simulink model "RL_TTS1_Controller_6E8X0_Ez_Test(9)"  (R2019b)
settings: Solver=VariableStepAuto  StartTime=0.0  StopTime=100  RelTol=1e-3
PostLoadFcn:
  | if any(exist('dsrtsu_mdlpostloadfcn', 'file') ~= 0), dsrtsu_mdlpostloadfcn('Execute', bdroot); end
undefined symbols (not defined in the file or in its folder): valve_position
libraries: simulink x5
settings Model: DSRTSU_INTERNAL_RTI_VER=550  DSRTSU_INTERNAL_RTI_TYPE=rti1104  RTICANMMDATA=struct('GeneralSetupData',struct('modelroot',['G:\RemoteLabs\RL git repos\Three Tank System set-up\dynamics-and-process-control-6e8x0\Teacher_files'],'generalsettings',struct('filesettings',struct('destfolder',struct('Name','RTICANMM_FILES','Check',1),'buildfolder',struct('Name','.','Check',1),'AbsDestfolder',struct('Name',['G:\RemoteLabs\RL git repos\Three Tank System set-up\dynamics-and-process-control-6e8x0\Teacher_files\RTICANMM_FILES']),'AbsBuildfolder',struct('Name',['G:\RemoteLabs\RL git repos\Three Tank System set-up\dynamics-and-process-control-6e8x0\Teacher_files']))),'options',struct('addpaths',1,'rmpaths',1,'addtrcexclusion',true,'cannavigator',struct('checkmonitoring',0),'show_usrtrc',0,'use_usrtrc',0),'advanced',struct('options',ones(1,100)),'MPSetup',{{}},'RTI',struct('Type','GRT','Ver','','Date',''),'modelname','RL_TTS1_Controller','block','RL_TTS1_Controller'))  DSRTSU_INTERNAL_RTIFPGA=150  Creator=whendrix  LastModifiedBy=20191255
settings SFSimCC: CustomCodeUndefinedFunction=UseInterfaceOnly

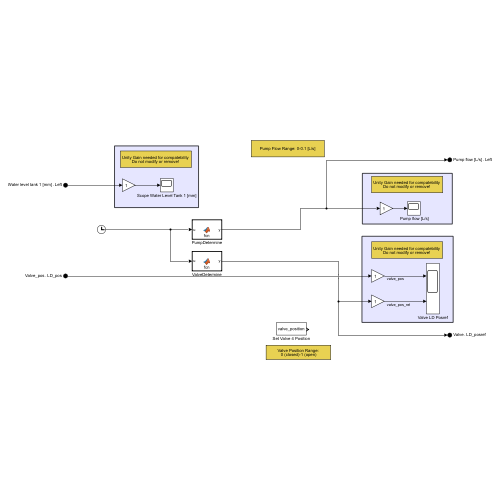
[thumbnail: Simulink's stored preview of the top-level diagram]
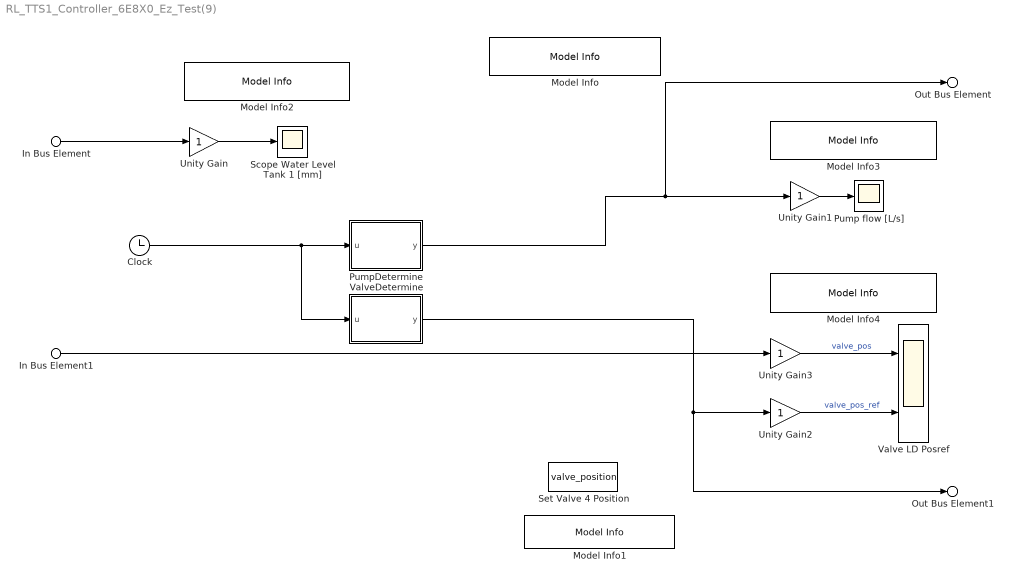
== system RL_TTS1_Controller_6E8X0_Ez_Test(9) ==
  In Bus Element : Inport  PortName=Water level tank 1 [mm]  Element=Left
  In Bus Element1 : Inport  Port=2  PortName=Valve_pos  Element=LD_pos
  " Pump flow [L/s]" : Scope
  Clock : Clock
  Model Info : simulink/Model-Wide Utilities/Model Info  Frame=on  DisplayStringWithTags=Pump Flow Range: 0-0.1 [L/s]  HorizontalTextAlignment=Center  LeftAlignmentValue=0.5
  Model Info1 : simulink/Model-Wide Utilities/Model Info  Frame=on  DisplayStringWithTags=|  HorizontalTextAlignment=Center  LeftAlignmentValue=0.5
      | Valve Position Range:
      |  0 (closed)-1 (open)
  Model Info2 : simulink/Model-Wide Utilities/Model Info  Frame=on  DisplayStringWithTags=Unity Gain needed for compatebility Do not modify or remove!  HorizontalTextAlignment=Center  LeftAlignmentValue=0.5
  Model Info3 : simulink/Model-Wide Utilities/Model Info  Frame=on  DisplayStringWithTags=Unity Gain needed for compatebility Do not modify or remove!  HorizontalTextAlignment=Center  LeftAlignmentValue=0.5
  Model Info4 : simulink/Model-Wide Utilities/Model Info  Frame=on  DisplayStringWithTags=Unity Gain needed for compatebility Do not modify or remove!  HorizontalTextAlignment=Center  LeftAlignmentValue=0.5
  PumpDetermine : MATLAB Function  TreatAsAtomicUnit=on
  Scope Water Level Tank 1 [mm] : Scope
  Set Valve 4 Position : Constant  Value=valve_position
  Unity Gain{,1..3} (4 alike) : Gain
  Valve LD Posref : Scope  NumInputPorts=2
  ValveDetermine : MATLAB Function  TreatAsAtomicUnit=on
  Out Bus Element : Outport  PortName=Pump flow [L/s]  Element=Left
  Out Bus Element1 : Outport  Port=2  PortName=Valve  Element=LD_posref
  wires:
  In Bus Element/1 -> Unity Gain/1
  Unity Gain/1 -> Scope Water Level Tank 1 [mm]/1
  Unity Gain1/1 -> " Pump flow [L/s]"/1
  Unity Gain3/1 -> Valve LD Posref/1  "valve_pos"
  In Bus Element1/1 -> Unity Gain3/1
  Unity Gain2/1 -> Valve LD Posref/2  "valve_pos_ref"
  Clock/1 -> ValveDetermine/1(u), PumpDetermine/1(u)
  ValveDetermine/1(y) -> Out Bus Element1/1, Unity Gain2/1
  PumpDetermine/1(y) -> Out Bus Element/1, Unity Gain1/1

== matlab function RL_TTS1_Controller_6E8X0_Ez_Test(9)/ValveDetermine ==
  data: u input; y output
function y = fcn(u)

y = ValveDetermine(u);

end

== matlab function RL_TTS1_Controller_6E8X0_Ez_Test(9)/PumpDetermine ==
  data: u input; y output
function y = fcn(u)

y = PumpDetermine(u);

end
